simulink model "P4_4"  (R2024b)
settings: Solver=VariableStepAuto  StartTime=0.0  StopTime=10  RelTol=1e-3
settings Model: Creator=Rj Avro Biswas  LastModifiedBy=Rj Avro Biswas

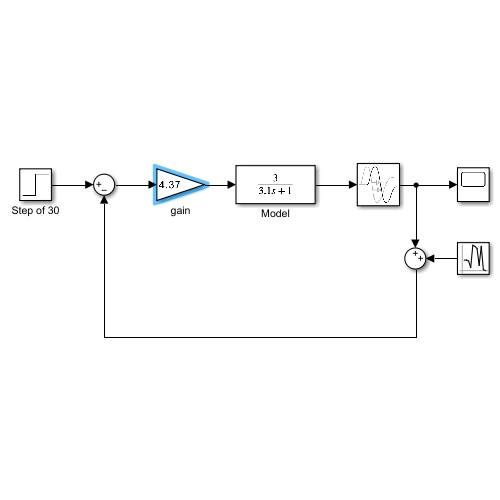
[thumbnail: Simulink's stored preview of the top-level diagram]
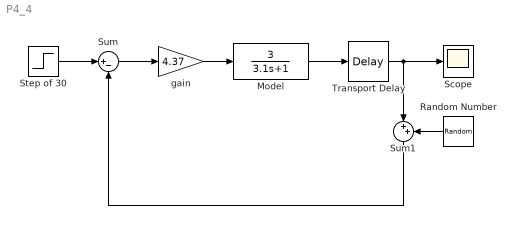
== system P4_4 ==
  Model : TransferFcn  Numerator=3  Denominator=[3.1 1]
  Random Number : RandomNumber  Variance=.5  Seed=61233  SampleTime=0
  Scope : Scope
  Step of 30 : Step  Time=0  After=30  SampleTime=0
  Sum : Sum  Inputs=|+-
  Sum1 : Sum  Inputs=|++
  Transport Delay : TransportDelay  DelayTime=0.15/60
  gain : Gain  Gain=4.37
  wires:
  Step of 30/1 -> Sum/1
  Sum/1 -> gain/1
  gain/1 -> Model/1
  Model/1 -> Transport Delay/1
  Transport Delay/1 -> Scope/1, Sum1/1
  Sum1/1 -> Sum/2
  Random Number/1 -> Sum1/2
